simulink model "Atomic_P_I"  (R2013b)
settings: Solver=FixedStepDiscrete  StartTime=0.0  StopTime=1  FixedStep=Te  RelTol=1e-3
values from neighbouring files (symbols this model uses):
  a0_pi = -1    [script.m]
  a0_s = 0.5488    [script.m]
  a1_pi = 1    [script.m]
  a1_s = -1.4816    [script.m]
  a2_s = 1    [script.m]
  b0_pi = -0.1750    (= -0.175)    [script.m]
  b0_s = 0.0302    [script.m]
  b1_pi = 0.25    [script.m]
  b1_s = 0.0369    [script.m]
  Te = 1e-4    (= 0.0001)    [script.m]
settings Model: TunableVars=Te,a0_pi,a0_s,a1_pi,a1_s,a2_s,b0_pi,b0_s,b1_pi,b1_s  TunableVarsStorageClass=Auto,Auto,Auto,Auto,Auto,Auto,Auto,Auto,Auto,Auto  TunableVarsTypeQualifier=,,,,,,,,,  Creator=gemsdev  LastModifiedBy=gemsdev
settings DataIOCC: ExternalInput=[t, x]  LoadExternalInput=on
settings OptimizationCC: InlineParams=on  OptimizeModelRefInitCode=on  LifeSpan=1
settings RTWCC: SystemTargetFile=ert.tlc  TemplateMakefile=RTW.MSVCBuild  Description=Create Visual C/C++ Solution File for Embedded Coder  ProcessScript=ert_make_rtw_hook  TargetLang=C++
settings CodeAppCC: IgnoreCustomStorageClasses=off
settings ERTTargetCC: CodeReplacementLibrary=ANSI_C  GenerateSampleERTMain=on  InlinedParameterPlacement=NonHierarchical  ERTCustomFileTemplate=example_file_process.tlc

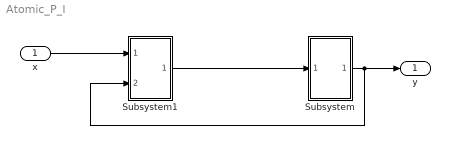
== system Atomic_P_I ==
  x : Inport
  Subsystem : Subsystem  TreatAsAtomicUnit=on  SystemSampleTime=Te
  Subsystem1 : Subsystem  TreatAsAtomicUnit=on  SystemSampleTime=Te
  y : Outport
  wires:
  Subsystem/1(Out1) -> y/1, Subsystem1/2(In2)
  x/1 -> Subsystem1/1(In1)
  Subsystem1/1(Out1) -> Subsystem/1(In1)

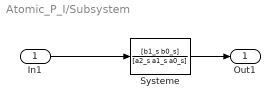
== system Atomic_P_I/Subsystem ==
  In1 : Inport
  Systeme : DiscreteTransferFcn  Numerator=[b1_s b0_s]  Denominator=[a2_s a1_s a0_s]  SampleTime=Te
  Out1 : Outport
  wires:
  Systeme/1 -> Out1/1
  In1/1 -> Systeme/1

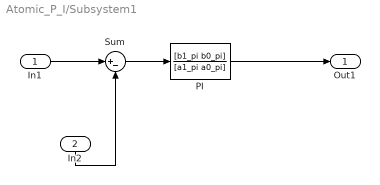
== system Atomic_P_I/Subsystem1 ==
  In1 : Inport
  In2 : Inport  Port=2
  PI : DiscreteTransferFcn  Numerator=[b1_pi b0_pi]  Denominator=[a1_pi a0_pi]  SampleTime=Te
  Sum : Sum  Inputs=|+-
  Out1 : Outport
  wires:
  Sum/1 -> PI/1
  In1/1 -> Sum/1
  In2/1 -> Sum/2
  PI/1 -> Out1/1
